simulink model "CCModel_73"  (R2024a)
settings: Solver=ode3  StartTime=0.0  StopTime=100  FixedStep=0.001  RelTol=1e-3  EnableMultiTasking=on
undefined symbols (not defined in the file or in its folder): DiscIntNeverNeededParam, Hecate_desVel1, Hecate_desVel2, Hecate_desVel3, Hecate_horShift, Hecate_period, Hecate_slope, Hecate_Transition1, Hecate_Transition2, Hecate_verShift, i, PME_qb, qb_map, RPM_qb, V
libraries: simulink x46
(part 1 of 11)
settings Model: Creator=user1  LastModifiedBy=fedformi_new
settings SolverCC: AlgebraicLoopSolver=TrustRegion
settings DataIOCC: SaveFormat=Array  SignalLoggingSaveFormat=ModelDataLogs  SignalLogging=off  DSMLogging=off
settings OptimizationCC: ReuseModelBlockBuffer=off  LifeSpan=inf
settings DebuggingCC: AlgebraicLoopMsg=none  FcnCallInpInsideContextMsg=warning  SFUnexpectedBacktrackingDiag=warning  SFNoUnconditionalDefaultTransitionDiag=warning  SFExecutionAtInitializationDiag=none  ArithmeticOperatorsInVariantConditions=warning
settings HardwareCC: ProdBitPerSizeT=32  ProdBitPerPtrDiffT=32  ProdWordSize=32  ProdHWDeviceType=Specified
settings ModelReferenceCC: EnableRefExpFcnMdlSchedulingChecks=on  PropagateSignalLabelsOutOfModel=off
settings SFSimCC: SimUseLocalCustomCode=off  CustomCodeUndefinedFunction=UseInterfaceOnly
settings RTWCC: RTWUseLocalCustomCode=off  GPUComputeCapability=3.5  DLArmComputeVersion=19.05
settings CodeAppCC: StateflowObjectComments=on
settings GRTTargetCC: TargetLangStandard=C89/C90 (ANSI)  CombineOutputUpdateFcns=off  GRTInterface=on
settings ConfigComp: CovMetricSettings=dw  CovSaveCumulativeToWorkspaceVar=on  CovSaveSingleToWorkspaceVar=on  CovExternalEMLEnable=off  DVTestSuiteOptimization=Auto  DVDetectOutOfBounds=on  DVModelReferenceHarness=on  DVHarnessSource=Signal Editor

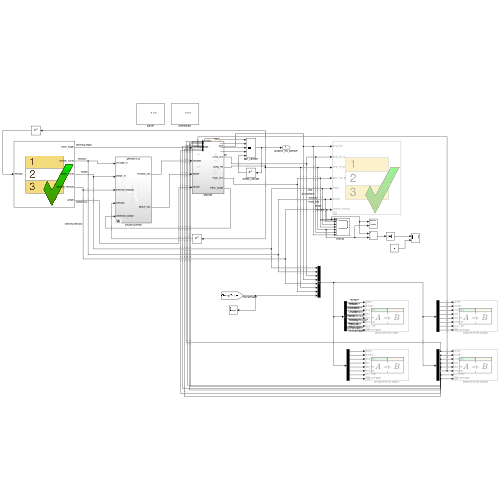
[thumbnail: Simulink's stored preview of the top-level diagram]
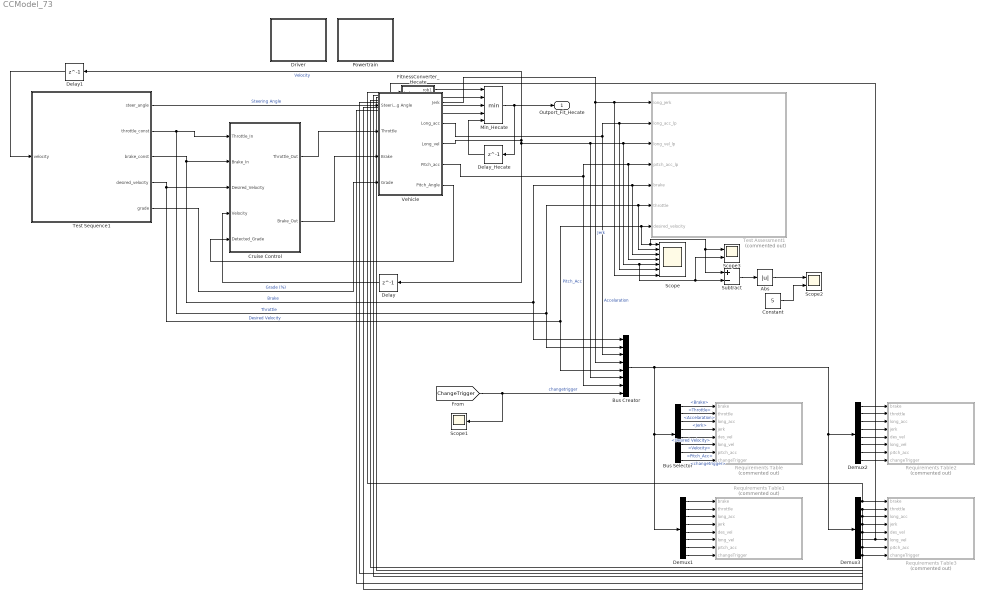
== system CCModel_73 ==
  Abs : Abs  SaturateOnIntegerOverflow=off
  Bus Creator : BusCreator  Inputs=8
  Bus Selector : BusSelector  OutputSignals=Brake,Throttle,Accelaration,Jerk,Desired Velocity,Velocity,Pitch_Acc,changetrigger
  Constant : Constant  Value=5
  Cruise Control : Subsystem  Variant=on  VariantControlMode=label  LabelModeActiveChoice=Version 7.3/7.4/7.5
  Delay : Delay  DelayLength=1
  Delay1 : Delay  DelayLength=1
  Delay_Hecate : Delay  DelayLength=1  InitialCondition=Inf
  Demux1 : Demux  Outputs=8
  Demux2 : Demux  Outputs=8
  Demux3 : Demux  Outputs=8
  Driver : Subsystem
      mask Display: image(imread('Driver_left.jpg'))
  FitnessConverter_Hecate : Stateflow chart  TreatAsAtomicUnit=on
  Min_Hecate : MinMax  Inputs=5
  Powertrain : Subsystem
      mask Display: image(imread('powertrain.jpg'))
  Requirements Table : Requirements Table  Commented=on  TreatAsAtomicUnit=on
  Requirements Table1 : Requirements Table  Commented=on  TreatAsAtomicUnit=on
  Requirements Table2 : Requirements Table  Commented=on  TreatAsAtomicUnit=on
  Requirements Table3 : Requirements Table  Commented=on  TreatAsAtomicUnit=on
  Scope : Scope  NumInputPorts=7
  Scope1 : Scope
  Scope2 : Scope  NumInputPorts=2
  Scope3 : Scope  NumInputPorts=2
  Subtract : Sum  Inputs=+-
  Test Assessment1 : Test Sequence  Commented=on  TreatAsAtomicUnit=on
  Test Sequence1 : Test Sequence  TreatAsAtomicUnit=on
  Vehicle : Subsystem
  Outport_Fit_Hecate : Outport
  wires:
  Test Sequence1/1(steer_angle) -> Vehicle/1(Steering Angle)  "Steering Angle"
  Test Sequence1/3(brake_const) -> Bus Creator/1, Scope/3, Test Assessment1/5(brake), Cruise Control/2(Brake_In)  "Brake"
  Test Sequence1/2(throttle_const) -> Bus Creator/2, Test Assessment1/6(throttle), Scope/2, Cruise Control/1(Throttle_In)  "Throttle"
  Test Sequence1/4(desired_velocity) -> Bus Creator/5, Subtract/1, Scope3/1, Scope/1, Test Assessment1/7(desired_velocity), Cruise Control/3(Desired_Velocity)  "Desired Velocity"
  Delay/1 -> Cruise Control/4(Velocity)
  Cruise Control/1(Throttle_Out) -> Vehicle/2(Throttle)
  Cruise Control/2(Brake_Out) -> Vehicle/3(Brake)
  Vehicle/4(Pitch_acc) -> Scope/4, Test Assessment1/4(pitch_acc_lp), Bus Creator/7  "Pitch_Acc"
  Vehicle/1(Jerk) -> Bus Creator/4, Scope/7, Test Assessment1/1(long_jerk)  "Jerk"
  Vehicle/2(Long_acc) -> Scope/6, Test Assessment1/2(long_acc_lp), Bus Creator/3  "Accelaration"
  Vehicle/3(Long_vel) -> Delay/1, Bus Creator/6, Scope3/2, Subtract/2, Scope/5, Test Assessment1/3(long_vel_lp), Delay1/1  "Velocity"
  Test Sequence1/5(grade) -> Vehicle/4(Grade)  "Grade (%)"
  Vehicle/5(Pitch_Angle) -> Cruise Control/5(Detected_Grade)
  Delay1/1 -> Test Sequence1/1(velocity)
  [ChangeTrigger] -> Bus Creator/8, Scope1/1  "changetrigger"
  Subtract/1 -> Abs/1
  Abs/1 -> Scope2/1
  Constant/1 -> Scope2/2
  Bus Selector/1 -> Requirements Table/1(brake)  "<Brake>"
  Bus Selector/2 -> Requirements Table/2(throttle)  "<Throttle>"
  Bus Selector/3 -> Requirements Table/3(long_acc)  "<Accelaration>"
  Bus Selector/4 -> Requirements Table/4(jerk)  "<Jerk>"
  Bus Selector/5 -> Requirements Table/5(des_vel)  "<Desired Velocity>"
  Bus Selector/6 -> Requirements Table/6(long_vel)  "<Velocity>"
  Bus Selector/7 -> Requirements Table/7(pitch_acc)  "<Pitch_Acc>"
  Bus Selector/8 -> Requirements Table/8(changeTrigger)  "<changetrigger>"
  Demux1/1 -> Requirements Table1/1(brake)
  Demux1/2 -> Requirements Table1/2(throttle)
  Demux1/3 -> Requirements Table1/3(long_acc)
  Demux1/4 -> Requirements Table1/4(jerk)
  Demux1/5 -> Requirements Table1/5(des_vel)
  Demux1/6 -> Requirements Table1/6(long_vel)
  Demux1/7 -> Requirements Table1/7(pitch_acc)
  Demux1/8 -> Requirements Table1/8(changeTrigger)
  Bus Creator/1 -> Demux1/1, Bus Selector/1, Demux3/1, Demux2/1
  Demux3/1 -> Requirements Table3/1(brake), FitnessConverter_Hecate/1(brake)
  Demux3/2 -> Requirements Table3/2(throttle), FitnessConverter_Hecate/2(throttle)
  Demux3/3 -> Requirements Table3/3(long_acc), FitnessConverter_Hecate/3(long_acc)
  Demux3/4 -> Requirements Table3/4(jerk), FitnessConverter_Hecate/4(jerk)
  Demux3/5 -> Requirements Table3/5(des_vel), FitnessConverter_Hecate/5(des_vel)
  Demux3/6 -> Requirements Table3/6(long_vel), FitnessConverter_Hecate/6(long_vel)
  Demux3/7 -> Requirements Table3/7(pitch_acc), FitnessConverter_Hecate/7(pitch_acc)
  Demux3/8 -> Requirements Table3/8(changeTrigger), FitnessConverter_Hecate/8(changeTrigger)
  Demux2/1 -> Requirements Table2/1(brake)
  Demux2/2 -> Requirements Table2/2(throttle)
  Demux2/3 -> Requirements Table2/3(long_acc)
  Demux2/4 -> Requirements Table2/4(jerk)
  Demux2/5 -> Requirements Table2/5(des_vel)
  Demux2/6 -> Requirements Table2/6(long_vel)
  Demux2/7 -> Requirements Table2/7(pitch_acc)
  Demux2/8 -> Requirements Table2/8(changeTrigger)
  FitnessConverter_Hecate/1(rob1) -> Min_Hecate/1
  FitnessConverter_Hecate/2(rob2) -> Min_Hecate/2
  FitnessConverter_Hecate/3(rob3) -> Min_Hecate/3
  FitnessConverter_Hecate/4(rob4) -> Min_Hecate/4
  Min_Hecate/1 -> Delay_Hecate/1, Outport_Fit_Hecate/1
  Delay_Hecate/1 -> Min_Hecate/5

== system CCModel_73/Cruise Control ==
  Throttle_In : Inport
  Brake_In : Inport  Port=2
  Desired_Velocity : Inport  Port=3
  Velocity : Inport  Port=4
  Detected_Grade : Inport  Port=5
  Version 1.0 : Subsystem  VariantControl=Version 1
  Version 2.0/2.1 : Subsystem  VariantControl=Version 2.0/2.1
  Version 3.0/3.1/3.2 : Subsystem  VariantControl=Version 3.0/3.1/3.2
  Version 4.0 : Subsystem  VariantControl=Version 4.0
  Version 5.0 : Subsystem  VariantControl=Version 5.0
  Version 6.0 : Subsystem  VariantControl=Version 6.0
  Version 6.1 : Subsystem  VariantControl=Version 6.1
  Version 6.2 : Subsystem  VariantControl=Version 6.2
  Version 6.3 : Subsystem  VariantControl=Version 6.3
  Version 6.4 : Subsystem  VariantControl=Version 6.4
  Version 6.5 : Subsystem  VariantControl=Version 6.5
  Version 6.6 : Subsystem  VariantControl=Version 6.6
  Version 7.0 : Subsystem  VariantControl=Version 7.0
  Version 7.1 : Subsystem  VariantControl=Version 7.1
  Version 7.2 : Subsystem  VariantControl=Version 7.2
  Version 7.3 : Subsystem  VariantControl=Version 7.3/7.4/7.5
  Throttle_Out : Outport
  Brake_Out : Outport  Port=2

== system CCModel_73/Driver ==
  Add : Sum  Inputs=+-
  Constant : Constant
  Gain3 : Gain  Gain=0.01
  Gain4 : Gain  Gain=0.01
  Manual Switch : ManualSwitch  CurrentSetting=0
  Memory3 : Memory
  Negative Motor Torque Table2 : Lookup_n-D  NumberOfTableDimensions=1  BreakpointsForDimension1="[5.65\t554.29\t1108.59\t1662.89\t2024.88\t2211.53\t2369.9\t2522.62\t2680.99\t2873.3\t3088.23\t3252.26\t3433.25\t3625.56\t3812.21\t4095.02\t4389.14\t4536.19\t4626.69\t4700.22\t4756.78\t4819\t4869.9\t4920.81\t4977.37\t4999.99]"  Table="[-444\t-444\t-444\t-444\t-428\t-416.41\t-396.47\t-372.36\t-344.93\t-310.84\t-285.92\t-268.48\t-248.55\t-233.62\t-218.68\t-200.45\t-193.05\t-186.44\t-173.14\t-154.84\t-129.037\t-101.56\t-73.26\t-46.62\t-17.48\t0]"  InternalRulePriority=Speed  RndMeth=Simplest
  Positive Motor Torque Table2 : Lookup_n-D  NumberOfTableDimensions=1  BreakpointsForDimension1=[1;10;575;750;925;1100;1275;1450;1625;1800;1975;2150;2325;2500;2675;2850;3025;3200;3375;3550;3725;3900;4075;4250;4425;4600;4775;4950;5125;5300;5475;5650;5825;6000]  Table=[412.5;412.5;412.5;412.5;412.5;412.5;412.5;412.5;412.5;412.5;412.5;412.5;412.5;412.5;412.5;412.5;412.5;412.5;412.5;412.5;400;380;355.5626875;346.30825;338.1746875;331.162;325.2701875;320.49925;316.8491875;314.32;308;275;50;0.195]  InternalRulePriority=Speed  RndMeth=Simplest
  Product : Product
  Product1 : Product
  Saturation : Saturate  UpperLimit=0  LowerLimit=-inf
  Saturation1 : Saturate  UpperLimit=inf  LowerLimit=0
  Scope1 : Scope
  Scope2 : Scope
  Switch : Switch  Criteria=u2 > Threshold  Threshold=0.05  SaturateOnIntegerOverflow=off  InputSameDT=off
  fd1 : Gain  Gain=3.87
  gb1 : Gain
  kph2mps1 : Gain  Gain=1/3.6
  rad_sec_to_rpm2 : Gain  Gain=9.55
  whl1 : Gain  Gain=1/0.3
  tag scope: Torque_Req=global
  wires:
  Switch/1 -> Scope1/1, Manual Switch/2
  Negative Motor Torque Table2/1 -> Product1/1
  Add/1 -> Gain4/1
  whl1/1 -> rad_sec_to_rpm2/1
  gb1/1 -> whl1/1
  [outVel] -> kph2mps1/1
  kph2mps1/1 -> fd1/1
  rad_sec_to_rpm2/1 -> Memory3/1
  Memory3/1 -> Negative Motor Torque Table2/1, Positive Motor Torque Table2/1
  Constant/1 -> Add/2
  fd1/1 -> gb1/1
  Gain3/1 -> Switch/2, Product/2
  Gain4/1 -> Product1/2
  Positive Motor Torque Table2/1 -> Product/1
  Product/1 -> Saturation1/1
  Product1/1 -> Saturation/1
  [throttle] -> Scope2/1, Gain3/1
  Saturation/1 -> Switch/3
  Saturation1/1 -> Switch/1
  [brake] -> Add/1
  Manual Switch/1 -> [Torque_Req]

== system CCModel_73/Powertrain ==
  note: Parallel Hybrid
  note: Electric
  note: Split Hybrid
  note: Conventional Powertrain
  note: Series Hybrid
  Brakes : Subsystem  Commented=on
      mask Display: image(imread('Brakes.jpg'))
  Central Differential : Subsystem  Commented=on  mask{CentralDifferentialActive=on, FrontBias=1}
      mask prompts: CentralDifferentialActive "Active"; FrontBias "Front Bias"
      mask Display: image(imread('differential.jpg'))
  Clutch : Subsystem  Commented=on  mask{ClutchActive=off}
      mask prompts: ClutchActive "Active"
      mask Display: image(imread('clutch.jpg'))
  EM0 : Subsystem  Commented=on  mask{EM0Active=off, EM0_Ratio=1}
      mask prompts: EM0Active "Active"; EM0_Ratio "Belt Ratio"
      mask Display: image(imread('Motor.jpg'))
  EM1 : Subsystem  Commented=on  mask{EM1Active=off, EM1_Ratio=1}
      mask prompts: EM1Active "Active"; EM1_Ratio "Conection Ratio"
      mask Display: image(imread('Motor.jpg'))
  EM2 : Subsystem  Commented=on  mask{EM2Active=off}
      mask prompts: EM2Active "Active"
      mask Display: image(imread('Motor.jpg'))
  EM3 : Subsystem  Commented=on  mask{EM3Active=off}
      mask prompts: EM3Active "Active"
      mask Display: image(imread('Motor.jpg'))
  EM4Front : Subsystem  Commented=on  mask{EM4FrontActive=off}
      mask prompts: EM4FrontActive "Active"
      mask Display: image(imread('Motor.jpg'))
  EM4Rear : Subsystem  Commented=on  mask{EM4RearActive=off}
      mask prompts: EM4RearActive "Active"
      mask Display: image(imread('Motor.jpg'))
  EMR : Subsystem  Commented=on  mask{EMRActive=off}
      mask prompts: EMRActive "Active"
      mask Display: image(imread('Motor.jpg'))
  EMS : Subsystem  Commented=on  mask{EMSActive=off}
      mask prompts: EMSActive "Active"
      mask Display: image(imread('Motor.jpg'))
  EV : Subsystem  mask{EVActive=on}
      mask prompts: EVActive "Active"
      mask Display: image(imread('Motor.jpg'))
  Engine : Subsystem  Commented=on  mask{EngineActive=off, IdleSpeed=0}
      mask prompts: EngineActive "Active"; IdleSpeed "Idle Speed (rpm)"
      mask Display: image(imread('engine.jpg'))
  Front Differential : Subsystem  Commented=on  mask{FrontDifferentialActive=on, DriveRatio=3.87}
      mask prompts: FrontDifferentialActive "Active"; DriveRatio "Drive Ratio"
      mask Display: image(imread('differential.jpg'))
  GEN : Subsystem  Commented=on  mask{GENActive=off}
      mask prompts: GENActive "Active"
      mask Display: image(imread('Motor.jpg'))
  Gearbox : Subsystem  Commented=on  mask{GearboxActive=off, AT=off}
      mask prompts: GearboxActive "Active"; AT "AT Active"
      mask Display: image(imread('gearbox.jpg'))
  MOT : Subsystem  Commented=on  mask{MOTActive=off}
      mask prompts: MOTActive "Active"
      mask Display: image(imread('Motor.jpg'))
  Rear Differential : Subsystem  Commented=on  mask{RearDifferentialActive=on, DriveRatio=1}
      mask prompts: RearDifferentialActive "Active"; DriveRatio "Drive Ratio"
      mask Display: image(imread('differential.jpg'))
  Split Device : Subsystem  Commented=on  mask{SplitActive=off, Ring2Sun=1}
      mask prompts: SplitActive "Active"; Ring2Sun "Ring to Sun Ratio"
      mask Display: image(imread('Motor.jpg'))

== system CCModel_73/Vehicle ==
  Steering Angle : Inport
  Throttle : Inport  Port=2
  Brake : Inport  Port=3
  Grade : Inport  Port=4
  Jerk : Outport
  Long_acc : Outport  Port=2
  Long_vel : Outport  Port=3
  Pitch_acc : Outport  Port=4
  Pitch_Angle : Outport  Port=5
  tag scope: outVel=global

== system CCModel_73/Cruise Control/Version 1.0 ==
  Throttle_In : Inport
  Brake_In : Inport  Port=2
  Desired_Velocity : Inport  Port=3
  Velocity : Inport  Port=4
  Inputs : Scope  NumInputPorts=2
  Manual Switch1 : ManualSwitch
  PID Controller : Subsystem
  Parameters : Scope  NumInputPorts=3
  Saturation1 : Saturate  UpperLimit=100  LowerLimit=0
  Saturation2 : Saturate  UpperLimit=100  LowerLimit=0
  Saturation3 : Saturate  UpperLimit=100  LowerLimit=0
  Sum2 : Sum  Inputs=|+-
  Throttle_Out : Outport
  Brake_Out : Outport  Port=2
  wires:
  Velocity/1 -> Sum2/2
  Saturation2/1 -> Brake_Out/1  "Brake"
  Manual Switch1/1 -> Throttle_Out/1  "throttle"
  Sum2/1 -> PID Controller/1(error)  "error"
  Saturation3/1 -> Manual Switch1/1, Inputs/2  "Throttle"
  Saturation1/1 -> Manual Switch1/2  "Throttle"
  PID Controller/1(u) -> Saturation3/1, Inputs/1  "u"
  Brake_In/1 -> Saturation2/1, Parameters/2  "Brake"
  Throttle_In/1 -> Parameters/1, Saturation1/1  "Throttle"
  Desired_Velocity/1 -> Sum2/1, Parameters/3  "Desired Velocity"

== system CCModel_73/Cruise Control/Version 2.0//2.1 ==
  Throttle_In : Inport
  Brake_In : Inport  Port=2
  Desired_Velocity : Inport  Port=3
  Velocity : Inport  Port=4
  Constant : Constant  Value=100
  Constant3 : Constant  Value=0
  Inputs : Scope  NumInputPorts=5
  Manual Switch{,1,3..4} (4 alike) : ManualSwitch
  PID Controller : Subsystem
  Parameters : Scope  NumInputPorts=4
  Saturation1 : Saturate  UpperLimit=100  LowerLimit=0
  Saturation2 : Saturate  UpperLimit=100  LowerLimit=0
  Sum2 : Sum  Inputs=|+-
  Switches : Subsystem
  Throttle_Out : Outport
  Brake_Out : Outport  Port=2
  wires:
  Manual Switch1/1 -> Manual Switch3/1  "throttle"
  Constant/1 -> Manual Switch3/2
  Switches/3(Source) -> Inputs/1  "Source"
  Manual Switch/1 -> Manual Switch4/1  "brake"
  Brake_In/1 -> Switches/3(brake_const), Saturation2/1, Parameters/3  "Brake"
  Switches/2(Brake) -> Manual Switch/1, Inputs/3  "Brake"
  Saturation1/1 -> Manual Switch1/2  "Throttle"
  Switches/1(Throttle) -> Manual Switch1/1, Inputs/2  "Throttle"
  Manual Switch4/1 -> Brake_Out/1
  Saturation2/1 -> Manual Switch/2  "Brake"
  Sum2/1 -> PID Controller/1(error)  "error"
  Desired_Velocity/1 -> Sum2/1, Parameters/4  "Desired Velocity"
  PID Controller/1(u) -> Switches/2(u), Inputs/4  "u"
  Constant3/1 -> Manual Switch4/2
  Manual Switch3/1 -> Throttle_Out/1
  Throttle_In/1 -> Switches/1(throttle_const), Parameters/2, Saturation1/1  "Throttle"
  Velocity/1 -> Sum2/2

== system CCModel_73/Cruise Control/Version 3.0//3.1//3.2 ==
  Throttle_In : Inport
  Brake_In : Inport  Port=2
  Desired_Velocity : Inport  Port=3
  Velocity : Inport  Port=4
  Add Constant : Bias  Bias=4  SaturateOnIntegerOverflow=off
  Detect Change : Subsystem
  Inputs : Scope  NumInputPorts=5
  Manual Switch : ManualSwitch
  Manual Switch1 : ManualSwitch
  PID Controller : Subsystem
  Parameters : Scope  NumInputPorts=4
  Saturation1 : Saturate  UpperLimit=100  LowerLimit=0
  Saturation2 : Saturate  UpperLimit=100  LowerLimit=0
  Saturation3 : Saturate  UpperLimit=100  LowerLimit=5
  Sum2 : Sum  Inputs=|+-
  Switches : Subsystem
  Throttle : Subsystem
  Throttle_Out : Outport
  Brake_Out : Outport  Port=2
  wires:
  Manual Switch1/1 -> Throttle_Out/1  "throttle"
  Switches/1(Throttle) -> Saturation3/1  "Throttle"
  Throttle/1(t_out) -> Switches/2(t_out)  "Smoothed u"
  Switches/2(Brake) -> Manual Switch/1, Inputs/3  "Brake"
  Saturation1/1 -> Manual Switch1/2  "Throttle"
  Sum2/1 -> PID Controller/1(error)  "error"
  Desired_Velocity/1 -> Add Constant/1, Parameters/4, Detect Change/1(desired_velocity)  "Desired Velocity"
  Switches/3(Source) -> Inputs/1  "Source"
  Throttle_In/1 -> Switches/1(throttle_const), Detect Change/2(throttle_const), Parameters/2, Saturation1/1  "Throttle"
  Manual Switch/1 -> Brake_Out/1  "brake"
  PID Controller/1(u) -> Inputs/4, Detect Change/4(u)  "u"
  Saturation2/1 -> Manual Switch/2  "Brake"
  Add Constant/1 -> Sum2/1
  Saturation3/1 -> Manual Switch1/1, Inputs/2  "Throttle"
  Brake_In/1 -> Switches/3(brake_const), Detect Change/3(brake_const), Saturation2/1, Parameters/3  "Brake"
  Detect Change/1(New u) -> Throttle/1(New u)
  Velocity/1 -> Sum2/2

== system CCModel_73/Cruise Control/Version 4.0 ==
  Throttle_In : Inport
  Brake_In : Inport  Port=2
  Desired_Velocity : Inport  Port=3
  Detected_Grade : Inport  Port=4
  Velocity : Inport  Port=5
  Abs : Abs  SaturateOnIntegerOverflow=off
  Delay : Delay  DelayLength=1
  Detect Change : Subsystem
  Inputs : Scope  NumInputPorts=5
  Outputs : Scope  NumInputPorts=4
  PID Controller : Subsystem
  Parameters : Scope  NumInputPorts=5
  Requirements : Scope  NumInputPorts=6
  Saturation1 : Saturate  UpperLimit=100  LowerLimit=-100
  Saturation2 : Saturate  UpperLimit=100  LowerLimit=-100
  Sigmoid : Subsystem
  Sum : Sum  Inputs=+-|
  Sum2 : Sum  Inputs=|+-
  Switches : Subsystem
  To Workspace4 : ToWorkspace  VariableName=steer_angle  SampleTime=-1
      settings: Save2DSignal=2-D array (concatenate along first dimension)
  To Workspace5 : ToWorkspace  VariableName=throttle  SampleTime=-1
      settings: Save2DSignal=2-D array (concatenate along first dimension)
  To Workspace8 : ToWorkspace  VariableName=brake  SampleTime=-1
      settings: Save2DSignal=2-D array (concatenate along first dimension)
  To Workspace9 : ToWorkspace  VariableName=vRef  SampleTime=-1
      settings: Save2DSignal=2-D array (concatenate along first dimension)
  Up CC Down Test : ManualSwitch
  Up CC Down Test 2 : ManualSwitch
  Throttle_Out : Outport
  Brake_Out : Outport  Port=2
  wires:
  [outVel] -> Sum/2, Requirements/1  "Velocity in km/hr"
  [longAcc] -> Requirements/2  "Acceleration in m/s^2"
  Sigmoid/1(u_out) -> Switches/2(u), Detect Change/4(Smoothed u), Inputs/5  "Smoothed u"
  Abs/1 -> Requirements/6  "Desired-Actual Velocity"
  [longAcc] -> Outputs/2  "Acceleration in m/s^2"
  Up CC Down Test/1 -> Brake_Out/1  "brake"
  [outVel] -> Outputs/3
  Desired_Velocity/1 -> Sum2/1, Detect Change/1(desired_velocity), To Workspace9/1, Parameters/4, [desired_velocity]  "Desired Velocity in km/hr"
  [jerk] -> Requirements/3
  Velocity/1 -> Delay/1
  Throttle_In/1 -> Saturation1/1  "Throttle"
  [brake] -> Outputs/1
  [pitchAcc] -> Requirements/4  "Pitch Acceleration in rad/s^2"
  Saturation1/1 -> [throttle], Parameters/2, To Workspace5/1, Up CC Down Test 2/2, Switches/1(throttle_const), Detect Change/2(throttle_const)  "Throttle"
  [desired_velocity] -> Sum/1, Requirements/5  "Desired Velocity in km/hr"
  Delay/1 -> Sum2/2
  Detect Change/3(hasChanged) -> Switches/4(hasChanged)
  Saturation2/1 -> Up CC Down Test/2, Switches/3(brake_const), Detect Change/3(brake_const), To Workspace8/1, Parameters/3, [brake]  "Brake"
  Sum/1 -> Abs/1
  Switches/1(Throttle) -> Up CC Down Test 2/1, Inputs/2  "Throttle"
  Switches/2(Brake) -> Up CC Down Test/1, Inputs/3  "Brake"
  PID Controller/1(u) -> Sigmoid/3(New u), Inputs/4  "u"
  Detected_Grade/1 -> Parameters/5  "Grade"
  Brake_In/1 -> Saturation2/1  "Brake"
  Switches/3(Source) -> Inputs/1  "Source"
  [desired_velocity] -> Outputs/4  "Desired Velocity in km/hr"
  Up CC Down Test 2/1 -> Throttle_Out/1  "throttle"
  Sum2/1 -> PID Controller/1(error)  "error"
  Detect Change/2(Old u) -> Sigmoid/2(Old u)
  Detect Change/1(Change_time) -> Sigmoid/1(Change_time)

== system CCModel_73/Cruise Control/Version 5.0 ==
  Throttle_In : Inport
  Brake_In : Inport  Port=2
  Desired_Velocity : Inport  Port=3
  Detected_Grade : Inport  Port=4
  Velocity : Inport  Port=5
  Abs : Abs  SaturateOnIntegerOverflow=off
  Delay : Delay  DelayLength=1
  Detect Change : Subsystem
  Inputs : Scope  NumInputPorts=5
  Outputs : Scope  NumInputPorts=4
  PID Controller : Subsystem
  Parameters : Scope  NumInputPorts=5
  Requirements : Scope  NumInputPorts=6
  Saturation1 : Saturate  UpperLimit=100  LowerLimit=-100
  Saturation2 : Saturate  UpperLimit=100  LowerLimit=-100
  Sigmoid : Subsystem
  Sum : Sum  Inputs=+-|
  Sum2 : Sum  Inputs=|+-
  Switches : Subsystem
  To Workspace4 : ToWorkspace  Commented=on  VariableName=steer_angle1  SampleTime=-1
      settings: Save2DSignal=2-D array (concatenate along first dimension)
  To Workspace5 : ToWorkspace  Commented=on  VariableName=throttle1  SampleTime=-1
      settings: Save2DSignal=2-D array (concatenate along first dimension)
  To Workspace8 : ToWorkspace  Commented=on  VariableName=brake1  SampleTime=-1
      settings: Save2DSignal=2-D array (concatenate along first dimension)
  To Workspace9 : ToWorkspace  Commented=on  VariableName=vRef1  SampleTime=-1
      settings: Save2DSignal=2-D array (concatenate along first dimension)
  Up CC Down Test : ManualSwitch
  Up CC Down Test 2 : ManualSwitch
  Throttle_Out : Outport
  Brake_Out : Outport  Port=2
  tag scope: brake=global
  wires:
  [jerk] -> Requirements/3  "Jerk"
  Switches/3(Source) -> Inputs/1  "Source"
  [outVel] -> Outputs/3
  Switches/2(Brake) -> Up CC Down Test/1, Inputs/3  "Brake"
  Up CC Down Test 2/1 -> Throttle_Out/1  "throttle"
  Throttle_In/1 -> Saturation1/1  "Throttle"
  [longAcc] -> Outputs/2  "Acceleration in m/s^2"
  Velocity/1 -> Delay/1
  Detect Change/3(hasChanged) -> Switches/4(hasChanged)
  Sigmoid/1(u_out) -> Switches/2(u), Detect Change/4(Smoothed u), Inputs/5  "Smoothed u"
  [outVel] -> Sum/2, Requirements/1  "Velocity in km/hr"
  [desired_velocity] -> Outputs/4  "Desired Velocity in km/hr"
  [desired_velocity] -> Sum/1, Requirements/5  "Desired Velocity in km/hr"
  Desired_Velocity/1 -> Sum2/1, To Workspace9/1, Parameters/4, [desired_velocity], Detect Change/1(desired_velocity)  "Desired Velocity in km/hr"
  Switches/1(Throttle) -> Up CC Down Test 2/1, Inputs/2  "Throttle"
  Sum/1 -> Abs/1
  Abs/1 -> Requirements/6  "Desired-Actual Velocity"
  PID Controller/1(u) -> Sigmoid/3(New u), Inputs/4  "u"
  Detect Change/1(Change_time) -> Sigmoid/1(Change_time)
  Brake_In/1 -> Saturation2/1  "Brake"
  Delay/1 -> Sum2/2
  [brake] -> Outputs/1
  Detect Change/2(Old u) -> Sigmoid/2(Old u)
  Saturation1/1 -> Up CC Down Test 2/2, Switches/1(throttle_const), Detect Change/2(throttle_const), Parameters/2, To Workspace5/1  "Throttle"
  Saturation2/1 -> Up CC Down Test/2, Switches/3(brake_const), Detect Change/3(brake_const), To Workspace8/1, Parameters/3, [brake]  "Brake"
  Sum2/1 -> PID Controller/1(error)  "error"
  Detected_Grade/1 -> Switches/5(Grade), PID Controller/2(Grade), Parameters/5  "Grade"
  [longAcc] -> Requirements/2  "Acceleration in m/s^2"
  [pitchAcc] -> Requirements/4  "Pitch Acceleration in rad/s^2"
  Up CC Down Test/1 -> Brake_Out/1  "brake"

== system CCModel_73/Cruise Control/Version 6.0 ==
  Throttle_In : Inport
  Brake_In : Inport  Port=2
  Desired_Velocity : Inport  Port=3
  Detected_Grade : Inport  Port=4
  Velocity : Inport  Port=5
  Abs : Abs  SaturateOnIntegerOverflow=off
  Detect Change : Subsystem
  Inputs : Scope  NumInputPorts=5
  Outputs : Scope  NumInputPorts=4
  PID Controller : Subsystem
  Parameters : Scope  NumInputPorts=5
  Requirements : Scope  NumInputPorts=6
  Saturation1 : Saturate  UpperLimit=100  LowerLimit=-100
  Saturation2 : Saturate  UpperLimit=100  LowerLimit=-100
  Sigmoid : Subsystem
  Sum : Sum  Inputs=+-|
  Sum2 : Sum  Inputs=|+-
  Switches : Subsystem
  To Workspace4 : ToWorkspace  Commented=on  VariableName=steer_angle2  SampleTime=-1
      settings: Save2DSignal=2-D array (concatenate along first dimension)
  To Workspace5 : ToWorkspace  Commented=on  VariableName=throttle2  SampleTime=-1
      settings: Save2DSignal=2-D array (concatenate along first dimension)
  To Workspace8 : ToWorkspace  Commented=on  VariableName=brake2  SampleTime=-1
      settings: Save2DSignal=2-D array (concatenate along first dimension)
  To Workspace9 : ToWorkspace  Commented=on  VariableName=vRef2  SampleTime=-1
      settings: Save2DSignal=2-D array (concatenate along first dimension)
  Up CC Down Test : ManualSwitch
  Up CC Down Test 2 : ManualSwitch
  Throttle_Out : Outport
  Brake_Out : Outport  Port=2
  tag scope: brake=global
  wires:
  [longAcc] -> Outputs/2  "Acceleration in m/s^2"
  [pitchAcc] -> Requirements/4  "Pitch Acceleration in rad/s^2"
  [desired_velocity] -> Outputs/4  "Desired Velocity in km/hr"
  [desired_velocity] -> Sum/1, Requirements/5  "Desired Velocity in km/hr"
  [outVel] -> Outputs/3
  Detect Change/3(hasChanged) -> Switches/4(hasChanged)
  Abs/1 -> Requirements/6  "Desired-Actual Velocity"
  Detect Change/2(Old u) -> Sigmoid/2(Old u)
  Switches/1(Throttle) -> Up CC Down Test 2/1, Inputs/2  "Throttle"
  Sum2/1 -> PID Controller/1(error)  "error"
  Detect Change/1(Change_time) -> Sigmoid/1(Change_time)
  Brake_In/1 -> Saturation2/1  "Brake"
  Saturation2/1 -> Up CC Down Test/2, Switches/3(brake_const), Detect Change/3(brake_const), To Workspace8/1, Parameters/3, [brake]  "Brake"
  Sum/1 -> Abs/1
  Throttle_In/1 -> Saturation1/1  "Throttle"
  [jerk] -> Requirements/3  "Jerk"
  Detected_Grade/1 -> PID Controller/2(Grade), Switches/5(Grade), Parameters/5
  [longAcc] -> Requirements/2  "Acceleration in m/s^2"
  Desired_Velocity/1 -> Sum2/1, To Workspace9/1, Parameters/4, [desired_velocity], Detect Change/1(desired_velocity)
  Up CC Down Test 2/1 -> Throttle_Out/1  "throttle"
  PID Controller/1(u) -> Sigmoid/3(New u), Inputs/4  "u"
  Velocity/1 -> Sum2/2
  Sigmoid/1(u_out) -> Switches/2(u), Detect Change/4(Smoothed u), Inputs/5  "Smoothed u"
  Saturation1/1 -> Up CC Down Test 2/2, Switches/1(throttle_const), Detect Change/2(throttle_const), [userThrottle], Parameters/2, To Workspace5/1  "Throttle"
  Switches/2(Brake) -> Up CC Down Test/1, Inputs/3  "Brake"
  [outVel] -> Sum/2, Requirements/1  "Velocity in km/hr"
  [brake] -> Outputs/1
  Switches/3(Source) -> Inputs/1  "Source"
  Up CC Down Test/1 -> Brake_Out/1  "brake"

== system CCModel_73/Cruise Control/Version 6.1 ==
  Throttle_In : Inport
  Brake_In : Inport  Port=2
  Desired_Velocity : Inport  Port=3
  Detected_Grade : Inport  Port=4
  Velocity : Inport  Port=5
  Abs : Abs  SaturateOnIntegerOverflow=off
  Delay : Delay  DelayLength=1
  Detect Change : Subsystem
  Inputs : Scope  NumInputPorts=5
  Outputs : Scope  NumInputPorts=4
  PID Controller : Subsystem
  Parameters : Scope  NumInputPorts=5
  Requirements : Scope  NumInputPorts=6
  Saturation1 : Saturate  UpperLimit=100  LowerLimit=-100
  Saturation2 : Saturate  UpperLimit=100  LowerLimit=-100
  Sigmoid : Subsystem
  Sum : Sum  Inputs=+-|
  Sum2 : Sum  Inputs=|+-
  Switches : Subsystem
  To Workspace4 : ToWorkspace  Commented=on  VariableName=steer_angle3  SampleTime=-1
      settings: Save2DSignal=2-D array (concatenate along first dimension)
  To Workspace5 : ToWorkspace  Commented=on  VariableName=throttle3  SampleTime=-1
      settings: Save2DSignal=2-D array (concatenate along first dimension)
  To Workspace8 : ToWorkspace  Commented=on  VariableName=brake3  SampleTime=-1
      settings: Save2DSignal=2-D array (concatenate along first dimension)
  To Workspace9 : ToWorkspace  Commented=on  VariableName=vRef3  SampleTime=-1
      settings: Save2DSignal=2-D array (concatenate along first dimension)
  Up CC Down Test : ManualSwitch
  Up CC Down Test 2 : ManualSwitch
  Throttle_Out : Outport
  Brake_Out : Outport  Port=2
  tag scope: ChangeTrigger=global, brake=global
  wires:
  Saturation1/1 -> Up CC Down Test 2/2, Switches/1(throttle_const), Detect Change/2(throttle_const), [userThrottle], Parameters/2, To Workspace5/1  "Throttle"
  [longAcc] -> Outputs/2  "Acceleration in m/s^2"
  PID Controller/2(P) -> Switches/6(P)
  Detect Change/3(hasChanged) -> [ChangeTrigger], Switches/4(hasChanged)
  Detect Change/1(Change_time) -> Sigmoid/1(Change_time)
  Sum/1 -> Abs/1
  Switches/2(Brake) -> Up CC Down Test/1, Inputs/3  "Brake"
  [pitchAcc] -> Requirements/4  "Pitch Acceleration in rad/s^2"
  [outVel] -> Outputs/3
  Brake_In/1 -> Saturation2/1  "Brake"
  [longAcc] -> Requirements/2  "Acceleration in m/s^2"
  Delay/1 -> Sum2/2
  [jerk] -> Requirements/3  "Jerk"
  Velocity/1 -> Delay/1
  [desired_velocity] -> Outputs/4  "Desired Velocity in km/hr"
  [desired_velocity] -> Sum/1, Requirements/5  "Desired Velocity in km/hr"
  Abs/1 -> Requirements/6  "Desired-Actual Velocity"
  Sigmoid/1(u_out) -> Switches/2(u), Detect Change/4(Smoothed u), Inputs/5  "Smoothed u"
  Up CC Down Test 2/1 -> Throttle_Out/1  "throttle"
  Detect Change/2(Old u) -> Sigmoid/2(Old u)
  [brake] -> Outputs/1
  [outVel] -> Sum/2, Requirements/1  "Velocity in km/hr"
  Switches/1(Throttle) -> Up CC Down Test 2/1, Inputs/2  "Throttle"
  PID Controller/1(u) -> Sigmoid/3(New u), Inputs/4  "u"
  Throttle_In/1 -> Saturation1/1  "Throttle"
  Switches/3(Source) -> Inputs/1  "Source"
  Saturation2/1 -> Up CC Down Test/2, Switches/3(brake_const), Detect Change/3(brake_const), To Workspace8/1, Parameters/3, [brake]  "Brake"
  Sum2/1 -> PID Controller/1(error)  "error"
  Detected_Grade/1 -> PID Controller/2(Grade), Switches/5(Grade)
  Desired_Velocity/1 -> Sum2/1, To Workspace9/1, Parameters/4, [desired_velocity], Detect Change/1(desired_velocity)  "Desired Velocity in km/hr"
  Up CC Down Test/1 -> Brake_Out/1  "brake"

== system CCModel_73/Cruise Control/Version 6.2 ==
  Throttle_In : Inport
  Brake_In : Inport  Port=2
  Desired_Velocity : Inport  Port=3
  Detected_Grade : Inport  Port=4
  Velocity : Inport  Port=5
  Abs : Abs  SaturateOnIntegerOverflow=off
  Detect Change : Subsystem
  Inputs : Scope  NumInputPorts=5
  Outputs : Scope  NumInputPorts=5
  PID Controller : Subsystem
  Parameters : Scope  NumInputPorts=5
  Requirements : Scope  NumInputPorts=6
  Saturation1 : Saturate  UpperLimit=100  LowerLimit=-100
  Saturation2 : Saturate  UpperLimit=100  LowerLimit=-100
  Sigmoid : Subsystem
  Sum : Sum  Inputs=+-|
  Sum2 : Sum  Inputs=|+-
  Switches : Subsystem
  To Workspace4 : ToWorkspace  Commented=on  VariableName=steer_angle4  SampleTime=-1
      settings: Save2DSignal=2-D array (concatenate along first dimension)
  To Workspace5 : ToWorkspace  Commented=on  VariableName=throttle4  SampleTime=-1
      settings: Save2DSignal=2-D array (concatenate along first dimension)
  To Workspace8 : ToWorkspace  Commented=on  VariableName=brake4  SampleTime=-1
      settings: Save2DSignal=2-D array (concatenate along first dimension)
  To Workspace9 : ToWorkspace  Commented=on  VariableName=vRef4  SampleTime=-1
      settings: Save2DSignal=2-D array (concatenate along first dimension)
  Up CC Down Test : ManualSwitch
  Up CC Down Test 2 : ManualSwitch
  Throttle_Out : Outport
  Brake_Out : Outport  Port=2
  tag scope: ChangeTrigger=global, brake=global
  wires:
  Saturation2/1 -> Up CC Down Test/2, Switches/3(brake_const), Detect Change/3(brake_const), To Workspace8/1, Parameters/3, [brake]  "Brake"
  Switches/3(Source) -> Inputs/1  "Source"
  Switches/1(Throttle) -> Up CC Down Test 2/1, Inputs/2  "Throttle"
  Throttle_In/1 -> Saturation1/1  "Throttle"
  Sigmoid/1(u_out) -> Switches/2(u), Detect Change/4(Smoothed u), Inputs/5  "Smoothed u"
  Brake_In/1 -> Saturation2/1  "Brake"
  [longAcc] -> Requirements/2  "Acceleration in m/s^2"
  [jerk] -> Requirements/3  "Jerk"
  [outVel] -> Outputs/4  "Actual Velocity in km/hr"
  [outVel] -> Sum/2, Requirements/1  "Velocity in km/hr"
  Sum2/1 -> PID Controller/1(error)  "error"
  Saturation1/1 -> Up CC Down Test 2/2, Switches/1(throttle_const), Detect Change/2(throttle_const), [userThrottle], Parameters/2, To Workspace5/1  "Throttle"
  [pitchAcc] -> Requirements/4  "Pitch Acceleration in rad/s^2"
  Switches/2(Brake) -> Up CC Down Test/1, Inputs/3  "Brake"
  Desired_Velocity/1 -> Sum2/1, To Workspace9/1, Parameters/4, [desired_velocity], Detect Change/1(desired_velocity)  "Desired Velocity in km/hr"
  [desired_velocity] -> Outputs/5  "Desired Velocity in km/hr"
  Sum/1 -> Abs/1
  Detect Change/2(Old u) -> Sigmoid/2(Old u)
  Detect Change/3(hasChanged) -> [ChangeTrigger], Switches/4(hasChanged)
  Abs/1 -> Requirements/6  "Desired-Actual Velocity"
  PID Controller/2(P) -> Switches/6(P)
  Detected_Grade/1 -> PID Controller/2(Grade), Switches/5(Grade)
  Detect Change/1(Change_time) -> Sigmoid/1(Change_time)
  PID Controller/1(u) -> Sigmoid/3(New u), Inputs/4  "u"
  Up CC Down Test 2/1 -> Throttle_Out/1  "throttle"
  [desired_velocity] -> Sum/1, Requirements/5  "Desired Velocity in km/hr"
  [longAcc] -> Outputs/2  "Acceleration in m/s^2"
  [jerk] -> Outputs/1  "Jerk"
  Velocity/1 -> Sum2/2
  Up CC Down Test/1 -> Brake_Out/1  "brake"

== system CCModel_73/Cruise Control/Version 6.3 ==
  Throttle_In : Inport
  Brake_In : Inport  Port=2
  Desired_Velocity : Inport  Port=3
  Detected_Grade : Inport  Port=4
  Velocity : Inport  Port=5
  Abs : Abs  SaturateOnIntegerOverflow=off
  Apply_Grade : Subsystem
  Detect Change : Subsystem
  Inputs : Scope  NumInputPorts=4
  Outputs : Scope  NumInputPorts=5
  PID Controller : Subsystem
  Parameters : Scope  NumInputPorts=5
  Requirements : Scope  NumInputPorts=6
  Saturation1 : Saturate  UpperLimit=100  LowerLimit=-100
  Saturation2 : Saturate  UpperLimit=100  LowerLimit=-100
  Sigmoid : Subsystem
  Sum : Sum  Inputs=+-|
  Sum2 : Sum  Inputs=|+-
  Switches : Subsystem
  To Workspace4 : ToWorkspace  Commented=on  VariableName=steer_angle5  SampleTime=-1
      settings: Save2DSignal=2-D array (concatenate along first dimension)
  To Workspace5 : ToWorkspace  Commented=on  VariableName=throttle5  SampleTime=-1
      settings: Save2DSignal=2-D array (concatenate along first dimension)
  To Workspace8 : ToWorkspace  Commented=on  VariableName=brake5  SampleTime=-1
      settings: Save2DSignal=2-D array (concatenate along first dimension)
  To Workspace9 : ToWorkspace  Commented=on  VariableName=vRef5  SampleTime=-1
      settings: Save2DSignal=2-D array (concatenate along first dimension)
  Up CC Down Test : ManualSwitch
  Up CC Down Test 2 : ManualSwitch
  Throttle_Out : Outport
  Brake_Out : Outport  Port=2
  tag scope: ChangeTrigger=global, brake=global
  wires:
  Throttle_In/1 -> Saturation1/1  "Throttle"
  Brake_In/1 -> Saturation2/1  "Brake"
  [longAcc] -> Requirements/2  "Acceleration in m/s^2"
  [jerk] -> Outputs/1  "Jerk"
  Detected_Grade/1 -> Apply_Grade/2(Grade), PID Controller/2(Grade)
  Up CC Down Test 2/1 -> Throttle_Out/1  "throttle"
  [jerk] -> Requirements/3  "Jerk"
  [outVel] -> Sum/2, Requirements/1  "Velocity in km/hr"
  [desired_velocity] -> Sum/1, Requirements/5  "Desired Velocity in km/hr"
  Velocity/1 -> Sum2/2
  [desired_velocity] -> Outputs/5  "Desired Velocity in km/hr"
  Abs/1 -> Requirements/6  "Desired-Actual Velocity"
  Switches/2(Brake) -> Up CC Down Test/1, Inputs/2  "Brake"
  Detect Change/1(Change_time) -> Sigmoid/3(Change_time)
  [pitchAcc] -> Requirements/4  "Pitch Acceleration in rad/s^2"
  Sigmoid/1(u_out) -> Switches/1(U), Detect Change/4(Smoothed u), Inputs/4  "Smoothed u"
  PID Controller/1(u) -> Apply_Grade/1(U_in)  "u"
  Saturation2/1 -> Switches/3(Brake_In), Up CC Down Test/2, Detect Change/3(brake_const), To Workspace8/1, Parameters/3, [brake]  "Brake"
  [longAcc] -> Outputs/2  "Acceleration in m/s^2"
  Switches/1(Throttle) -> Up CC Down Test 2/1, Inputs/1  "Throttle"
  Apply_Grade/1(U_Out) -> Sigmoid/2(U2), Inputs/3
  Desired_Velocity/1 -> To Workspace9/1, Parameters/4, [desired_velocity], Detect Change/1(desired_velocity), Sum2/1  "Desired Velocity in km/hr"
  [outVel] -> Outputs/4  "Actual Velocity in km/hr"
  Sum/1 -> Abs/1
  Sum2/1 -> PID Controller/1(error)  "error"
  Saturation1/1 -> Switches/2(Throttle_In), Up CC Down Test 2/2, Detect Change/2(throttle_const), [userThrottle], Parameters/2, To Workspace5/1  "Throttle"
  Detect Change/2(Old u) -> Sigmoid/1(U1)
  Up CC Down Test/1 -> Brake_Out/1  "brake"
  Detect Change/3(hasChanged) -> [ChangeTrigger]  "Source"

== system CCModel_73/Cruise Control/Version 6.4 ==
  Throttle_In : Inport
  Brake_In : Inport  Port=2
  Desired_Velocity : Inport  Port=3
  Detected_Grade : Inport  Port=4
  Velocity : Inport  Port=5
  Abs : Abs  SaturateOnIntegerOverflow=off
  Apply_Grade : Subsystem
  Detect Change : Subsystem
  Inputs : Scope  NumInputPorts=4
  Outputs : Scope  NumInputPorts=5
  PID Controller : Subsystem
  Parameters : Scope  NumInputPorts=5
  Requirements : Scope  NumInputPorts=6
  Saturation1 : Saturate  UpperLimit=100  LowerLimit=-100
  Saturation2 : Saturate  UpperLimit=100  LowerLimit=-100
  Sigmoid : Subsystem
  Sum : Sum  Inputs=+-|
  Sum2 : Sum  Inputs=|+-
  Switches : Subsystem
  To Workspace4 : ToWorkspace  Commented=on  VariableName=steer_angle6  SampleTime=-1
      settings: Save2DSignal=2-D array (concatenate along first dimension)
  To Workspace5 : ToWorkspace  Commented=on  VariableName=throttle6  SampleTime=-1
      settings: Save2DSignal=2-D array (concatenate along first dimension)
  To Workspace8 : ToWorkspace  Commented=on  VariableName=brake6  SampleTime=-1
      settings: Save2DSignal=2-D array (concatenate along first dimension)
  To Workspace9 : ToWorkspace  Commented=on  VariableName=vRef6  SampleTime=-1
      settings: Save2DSignal=2-D array (concatenate along first dimension)
  Up CC Down Test : ManualSwitch
  Up CC Down Test 2 : ManualSwitch
  Throttle_Out : Outport
  Brake_Out : Outport  Port=2
  tag scope: brake=global
  wires:
  [desired_velocity] -> Sum/1, Requirements/5  "Desired Velocity in km/hr"
  [outVel] -> Sum/2, Requirements/1  "Velocity in km/hr"
  Detect Change/2(Old u) -> Sigmoid/1(U1)
  ? -> ?
  Throttle_In/1 -> Saturation1/1  "Throttle"
  PID Controller/1(u) -> Apply_Grade/1(U_in)  "u"
  [jerk] -> Outputs/1  "Jerk"
  Detected_Grade/1 -> Apply_Grade/2(Grade), PID Controller/2(Grade)
  Detect Change/1(Change_time) -> Sigmoid/3(Change_time)
  [jerk] -> Requirements/3  "Jerk"
  [longAcc] -> Outputs/2  "Acceleration in m/s^2"
  Up CC Down Test 2/1 -> Throttle_Out/1  "throttle"
  Desired_Velocity/1 -> To Workspace9/1, Parameters/4, [desired_velocity], Detect Change/1(desired_velocity), Sum2/1  "Desired Velocity in km/hr"
  ? -> Parameters/1, To Workspace4/1  "Steering Angle"
  Sigmoid/1(u_out) -> Switches/1(U), Detect Change/4(Smoothed u), Inputs/4  "Smoothed u"
  Brake_In/1 -> Saturation2/1  "Brake"
  [outVel] -> Outputs/4  "Actual Velocity in km/hr"
  Apply_Grade/1(U_Out) -> Inputs/3, Sigmoid/2(U2)
  [pitchAcc] -> Requirements/4  "Pitch Acceleration in rad/s^2"
  Velocity/1 -> Sum2/2
  Abs/1 -> Requirements/6  "Desired-Actual Velocity"
  Switches/1(Throttle) -> Up CC Down Test 2/1, Inputs/1  "Throttle"
  [longAcc] -> Requirements/2  "Acceleration in m/s^2"
  Saturation1/1 -> Switches/2(Throttle_In), Up CC Down Test 2/2, Detect Change/2(throttle_const), [userThrottle], Parameters/2, To Workspace5/1  "Throttle"
  [desired_velocity] -> Outputs/5  "Desired Velocity in km/hr"
  Sum/1 -> Abs/1
  Switches/2(Brake) -> Inputs/2, Up CC Down Test/1  "Brake"
  Sum2/1 -> PID Controller/1(error)  "error"
  Saturation2/1 -> Switches/3(Brake_In), Up CC Down Test/2, Detect Change/3(brake_const), To Workspace8/1, Parameters/3, [brake]  "Brake"
  Up CC Down Test/1 -> Brake_Out/1  "brake"

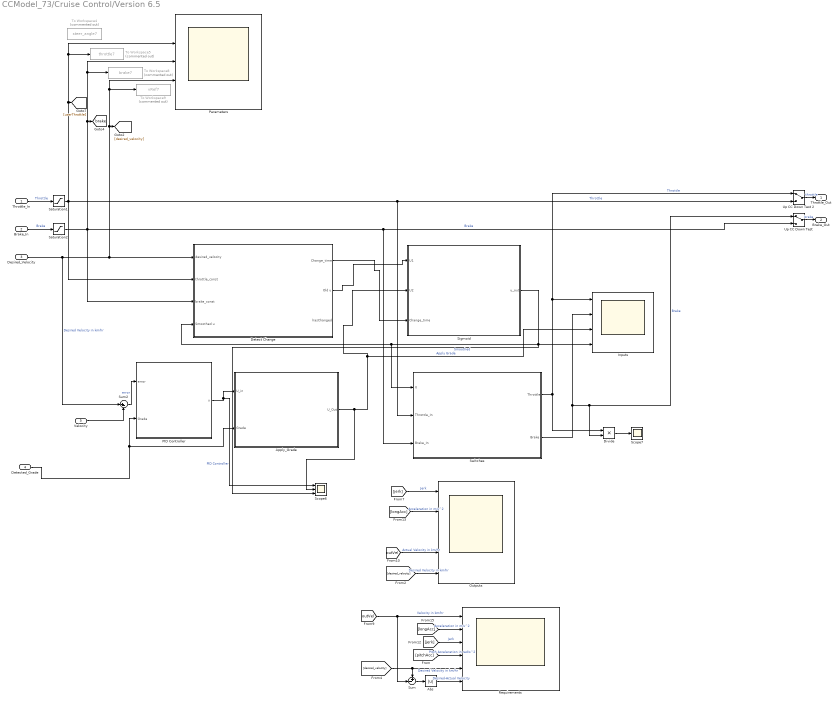
== system CCModel_73/Cruise Control/Version 6.5 ==
  Throttle_In : Inport
  Brake_In : Inport  Port=2
  Desired_Velocity : Inport  Port=3
  Detected_Grade : Inport  Port=4
  Velocity : Inport  Port=5
  Abs : Abs  SaturateOnIntegerOverflow=off
  Apply_Grade : Subsystem
  Detect Change : Subsystem
  Divide : Product  Inputs=**
  Inputs : Scope  NumInputPorts=4
  Outputs : Scope  NumInputPorts=5
  PID Controller : Subsystem
  Parameters : Scope  NumInputPorts=5
  Requirements : Scope  NumInputPorts=6
  Saturation1 : Saturate  UpperLimit=100  LowerLimit=-100
  Saturation2 : Saturate  UpperLimit=100  LowerLimit=-100
  Scope6 : Scope  NumInputPorts=3
  Scope7 : Scope
  Sigmoid : Subsystem
  Sum : Sum  Inputs=+-|
  Sum2 : Sum  Inputs=|+-
  Switches : Subsystem
  To Workspace4 : ToWorkspace  Commented=on  VariableName=steer_angle7  SampleTime=-1
      settings: Save2DSignal=2-D array (concatenate along first dimension)
  To Workspace5 : ToWorkspace  Commented=on  VariableName=throttle7  SampleTime=-1
      settings: Save2DSignal=2-D array (concatenate along first dimension)
  To Workspace8 : ToWorkspace  Commented=on  VariableName=brake7  SampleTime=-1
      settings: Save2DSignal=2-D array (concatenate along first dimension)
  To Workspace9 : ToWorkspace  Commented=on  VariableName=vRef7  SampleTime=-1
      settings: Save2DSignal=2-D array (concatenate along first dimension)
  Up CC Down Test : ManualSwitch
  Up CC Down Test 2 : ManualSwitch
  Throttle_Out : Outport
  Brake_Out : Outport  Port=2
  tag scope: brake=global
  wires:
  Throttle_In/1 -> Saturation1/1  "Throttle"
  Velocity/1 -> Sum2/2
  ? -> ?
  Divide/1 -> Scope7/1
  PID Controller/1(u) -> Scope6/1, Apply_Grade/1(U_in)  "PID Controller"
  [outVel] -> Sum/2, Requirements/1  "Velocity in km/hr"
  Sigmoid/1(u_out) -> Scope6/3, Switches/1(U), Detect Change/4(Smoothed u), Inputs/4  "Smoothed"
  Apply_Grade/1(U_Out) -> Scope6/2, Inputs/3, Sigmoid/2(U2)  "Apply Grade"
  Saturation2/1 -> Switches/3(Brake_In), Up CC Down Test/2, Detect Change/3(brake_const), To Workspace8/1, Parameters/3, [brake]  "Brake"
  [jerk] -> Outputs/1  "Jerk"
  Detected_Grade/1 -> Apply_Grade/2(Grade), PID Controller/2(Grade)
  Up CC Down Test 2/1 -> Throttle_Out/1  "throttle"
  [jerk] -> Requirements/3  "Jerk"
  [longAcc] -> Requirements/2  "Acceleration in m/s^2"
  Brake_In/1 -> Saturation2/1  "Brake"
  [pitchAcc] -> Requirements/4  "Pitch Acceleration in rad/s^2"
  [outVel] -> Outputs/4  "Actual Velocity in km/hr"
  [desired_velocity] -> Outputs/5  "Desired Velocity in km/hr"
  [desired_velocity] -> Sum/1, Requirements/5  "Desired Velocity in km/hr"
  Sum/1 -> Abs/1
  Detect Change/1(Change_time) -> Sigmoid/3(Change_time)
  Switches/2(Brake) -> Inputs/2, Divide/2, Up CC Down Test/1  "Brake"
  Abs/1 -> Requirements/6  "Desired-Actual Velocity"
  Desired_Velocity/1 -> To Workspace9/1, Parameters/4, [desired_velocity], Detect Change/1(desired_velocity), Sum2/1  "Desired Velocity in km/hr"
  Saturation1/1 -> Switches/2(Throttle_In), Up CC Down Test 2/2, Detect Change/2(throttle_const), [userThrottle], Parameters/2, To Workspace5/1  "Throttle"
  Detect Change/2(Old u) -> Sigmoid/1(U1)
  [longAcc] -> Outputs/2  "Acceleration in m/s^2"
  Sum2/1 -> PID Controller/1(error)  "error"
  Switches/1(Throttle) -> Up CC Down Test 2/1, Inputs/1, Divide/1  "Throttle"
  Up CC Down Test/1 -> Brake_Out/1  "brake"

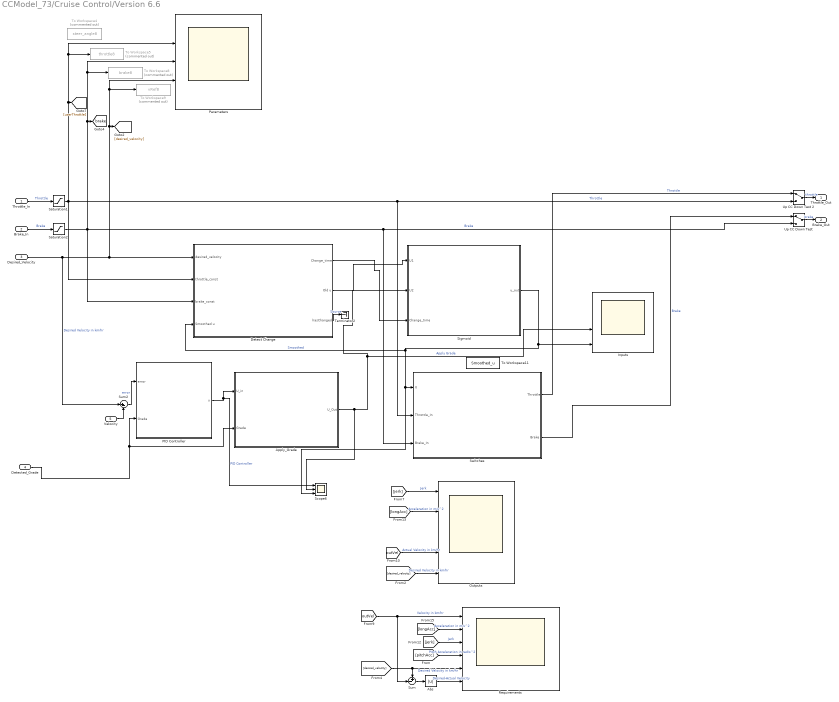
== system CCModel_73/Cruise Control/Version 6.6 ==
  Throttle_In : Inport
  Brake_In : Inport  Port=2
  Desired_Velocity : Inport  Port=3
  Detected_Grade : Inport  Port=4
  Velocity : Inport  Port=5
  Abs : Abs  SaturateOnIntegerOverflow=off
  Apply_Grade : Subsystem
  Detect Change : Subsystem
  Inputs : Scope  NumInputPorts=4
  Outputs : Scope  NumInputPorts=5
  PID Controller : Subsystem
  Parameters : Scope  NumInputPorts=5
  Requirements : Scope  NumInputPorts=6
  Saturation1 : Saturate  UpperLimit=100  LowerLimit=-100
  Saturation2 : Saturate  UpperLimit=100  LowerLimit=-100
  Scope6 : Scope  NumInputPorts=3
  Sigmoid : Subsystem
  Sum : Sum  Inputs=+-|
  Sum2 : Sum  Inputs=|+-
  Switches : Subsystem
  Terminator2 : Terminator
  To Workspace11 : ToWorkspace  VariableName=Smoothed_u  SampleTime=-1
  To Workspace4 : ToWorkspace  Commented=on  VariableName=steer_angle8  SampleTime=-1
      settings: Save2DSignal=2-D array (concatenate along first dimension)
  To Workspace5 : ToWorkspace  Commented=on  VariableName=throttle8  SampleTime=-1
      settings: Save2DSignal=2-D array (concatenate along first dimension)
  To Workspace8 : ToWorkspace  Commented=on  VariableName=brake8  SampleTime=-1
      settings: Save2DSignal=2-D array (concatenate along first dimension)
  To Workspace9 : ToWorkspace  Commented=on  VariableName=vRef8  SampleTime=-1
      settings: Save2DSignal=2-D array (concatenate along first dimension)
  Up CC Down Test : ManualSwitch
  Up CC Down Test 2 : ManualSwitch
  Throttle_Out : Outport
  Brake_Out : Outport  Port=2
  tag scope: brake=global
  wires:
  [desired_velocity] -> Sum/1, Requirements/5  "Desired Velocity in km/hr"
  [longAcc] -> Requirements/2  "Acceleration in m/s^2"
  [desired_velocity] -> Outputs/5  "Desired Velocity in km/hr"
  Abs/1 -> Requirements/6  "Desired-Actual Velocity"
  Saturation2/1 -> Switches/3(Brake_In), Up CC Down Test/2, Detect Change/3(brake_const), To Workspace8/1, Parameters/3, [brake]  "Brake"
  Desired_Velocity/1 -> To Workspace9/1, Parameters/4, [desired_velocity], Detect Change/1(desired_velocity), Sum2/1  "Desired Velocity in km/hr"
  Switches/2(Brake) -> Up CC Down Test/1  "Brake"
  Detect Change/1(Change_time) -> Sigmoid/3(Change_time)
  Throttle_In/1 -> Saturation1/1  "Throttle"
  Brake_In/1 -> Saturation2/1  "Brake"
  Detect Change/2(Old u) -> Sigmoid/1(U1)
  PID Controller/1(u) -> Scope6/1, Apply_Grade/1(U_in)  "PID Controller"
  [jerk] -> Outputs/1  "Jerk"
  Velocity/1 -> Sum2/2
  Sum/1 -> Abs/1
  Switches/1(Throttle) -> Up CC Down Test 2/1  "Throttle"
  [outVel] -> Sum/2, Requirements/1  "Velocity in km/hr"
  Detected_Grade/1 -> Apply_Grade/2(Grade), PID Controller/2(Grade)
  Saturation1/1 -> Switches/2(Throttle_In), Up CC Down Test 2/2, Detect Change/2(throttle_const), [userThrottle], Parameters/2, To Workspace5/1  "Throttle"
  [longAcc] -> Outputs/2  "Acceleration in m/s^2"
  [pitchAcc] -> Requirements/4  "Pitch Acceleration in rad/s^2"
  Sigmoid/1(u_out) -> Detect Change/4(Smoothed u), Scope6/3, Switches/1(U), Inputs/4  "Smoothed"
  Sum2/1 -> PID Controller/1(error)  "error"
  Apply_Grade/1(U_Out) -> Scope6/2, Inputs/3, Sigmoid/2(U2)  "Apply Grade"
  [jerk] -> Requirements/3  "Jerk"
  Up CC Down Test 2/1 -> Throttle_Out/1  "throttle"
  [outVel] -> Outputs/4  "Actual Velocity in km/hr"
  Detect Change/3(hasChanged) -> Terminator2/1  "Source"
  Up CC Down Test/1 -> Brake_Out/1  "brake"
